simulink model "tdm_test"  (R2015a)
settings: Solver=ode45  StartTime=0.0  StopTime=100.0  RelTol=1e-3
libraries: xbsIndex_r4 x9, simulink x1
settings Model: Creator=ACS  LastModifiedBy=ACS

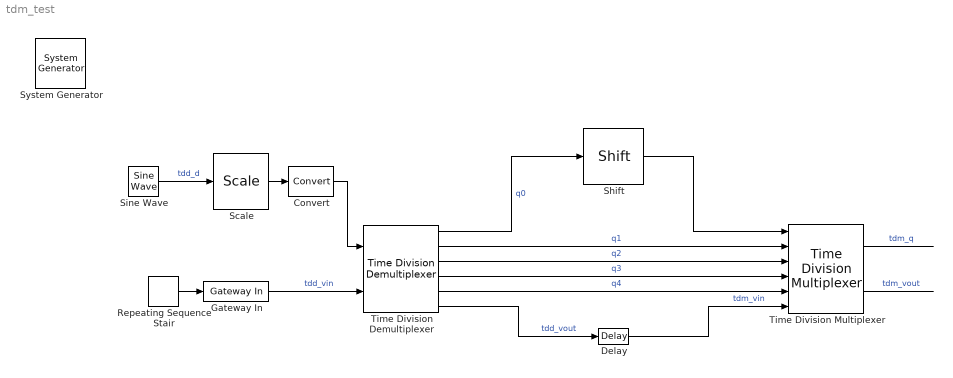
== system tdm_test ==
  " System Generator" : xbsIndex_r4/ System Generator  Tag=genX  xilinxfamily=virtex7  part=xc7vx485t  speed=-2  package=ffg1157  synthesis_tool=Vivado  clock_wrapper=Clock Enables  directory=./netlist  proj_type=Vivado  Synth_file=Vivado Synthesis Defaults  Impl_file=Vivado Implementation Defaults  testbench=off  simulink_period=1  sysclk_period=10  dcm_input_clock_period=10  incr_netlist=off  trim_vbits=Everywhere in SubSystem  dbl_ovrd=According to Block Masks  core_generation=According to Block Masks  run_coregen=off  deprecated_control=off  eval_field=0  block_type=sysgen
  Convert : xbsIndex_r4/Convert  gui_display_data_type=Fixed-point  arith_type="Signed  (2's comp)"  n_bits=15  bin_pt=0  float_type=Single  exp_bits=8  fraction_bits=24  quantization=Truncate  overflow=Wrap  en=off  latency=0  pipeline=off  dbl_ovrd=off  block_type=convert
  Delay : xbsIndex_r4/Delay  rst=off  infoeditControl=Selection of Reset will increase slice count due to use of real FFs and instead of SRLs  en=off  latency=1  reg_retiming=off  dbl_ovrd=off  block_type=delay
  Gateway In : xbsIndex_r4/Gateway In  gui_display_data_type=Boolean  arith_type=Boolean  n_bits=16  bin_pt=14  preci_type=Single  exp_width=8  frac_width=24  rows=1  columns=1  quantization="Round  (unbiased: +/- Inf)"  overflow=Saturate  period=1  UseAsADC=off  ADCChannel='1'  interface=None  automatic_assignment=on  address_offset=hex2dec('00')  intf_name=''  intf_description=''  timing_constraint=None  locs_specified=off  LOCs={}  io_standard={}  inherit_from_input=off  hdl_port=on  dbl_ovrd=off  block_type=gatewayin
  Repeating Sequence Stair : simulink/Sources/Repeating Sequence Stair  OutValues="[ 1 1 1 1 1 0 0 0 0 0  ].'"  tsamp=1  OutMin=[]  OutMax=[]  OutDataTypeStr=boolean  OutputDataTypeScalingMode=Specify via dialog  OutDataType=fixdt('boolean')  ConRadixGroup=Best Precision: Vector-wise  OutScaling=[]
  Scale : xbsIndex_r4/Scale  scale_factor=12  dbl_ovrd=off  block_type=scale
  Shift : xbsIndex_r4/Shift  shift_dir=Left  shift_bits=2  en=off  latency=1  precision=User Defined  arith_type="Signed  (2's comp)"  n_bits=15  bin_pt=0  quantization=Truncate  overflow=Wrap  dbl_ovrd=off  block_type=shift
  Sine Wave : xbsIndex_r4/Sine Wave  Input_format=Radians  output_frequency=0.5  phase_offset_angles=0  output_selection=Sine  sfdr=90  explicit_period=off  period=1  simulation_type=fast_sim  simulation_model=sysgen:dds_macro  block_type=dds_macro
  Time Division Demultiplexer : xbsIndex_r4/Time Division Demultiplexer  frame_pattern=[1 1 1 1 1]  impl_style=Multiple Channel  vin=on  explicit_period=off  dbl_ovrd=off  period=1  block_type=tdd
      settings: infoedit=Samples presented at the input are selected and down-sampled according to the frame sampling pattern specified. The sampled input is presented either as a single or multiple channel at the output.
  Time Division Multiplexer : xbsIndex_r4/Time Division Multiplexer  inputs=5  vin=on  Optimization=Resource  explicit_period=off  period=1  dbl_ovrd=off  block_type=tdm
      settings: infoedit="Multiple inputs are sampled and  presented serially at the output."
  wires:
  Sine Wave/1 -> Scale/1  "tdd_d"
  Repeating Sequence Stair/1 -> Gateway In/1
  Gateway In/1 -> Time Division Demultiplexer/2  "tdd_vin"
  Time Division Multiplexer/1 -> ?  "tdm_q"
  Time Division Multiplexer/2 -> ?  "tdm_vout"
  Time Division Demultiplexer/2 -> Time Division Multiplexer/2  "q1"
  Time Division Demultiplexer/5 -> Time Division Multiplexer/5  "q4"
  Time Division Demultiplexer/3 -> Time Division Multiplexer/3  "q2"
  Time Division Demultiplexer/4 -> Time Division Multiplexer/4  "q3"
  Time Division Demultiplexer/1 -> Shift/1  "q0"
  Shift/1 -> Time Division Multiplexer/1
  Delay/1 -> Time Division Multiplexer/6  "tdm_vin"
  Time Division Demultiplexer/6 -> Delay/1  "tdd_vout"
  Convert/1 -> Time Division Demultiplexer/1
  Scale/1 -> Convert/1
